simulink model "cranePoleMDL"  (R2014a)
settings: Solver=ode45  StartTime=0.0  StopTime=10.0  RelTol=1e-3
values from neighbouring files (symbols this model uses):
  F = A1-K1*C    [cartPole.m]    (also in chenEx3p3p3.m = A1-k1*C)
  g = 9.8    [cartPole.m]
  K = K1 + F*H    [cartPole.m]
  l = 0.3    [cartPole.m]
  M = .5    (= 0.5)    [cartPole.m]
  m = .2    (= 0.2)    [cartPole.m]
  theta_0 = pi    (= 3.14159265359)    [cartPole.m]
  theta_d_0 = 0.0    (= 0)    [cartPole.m]
  x1_0 = -1    [chenEx3p3p3.m]
  x3_0 = 1    [chenEx3p3p3.m]
  x_0 = 0    [cartPole.m]
  x_d_0 = 0    [cartPole.m]
undefined symbols (not defined in the file or in its folder): Klqr
settings Model: Creator=sqn4594  LastModifiedBy=sqn4594

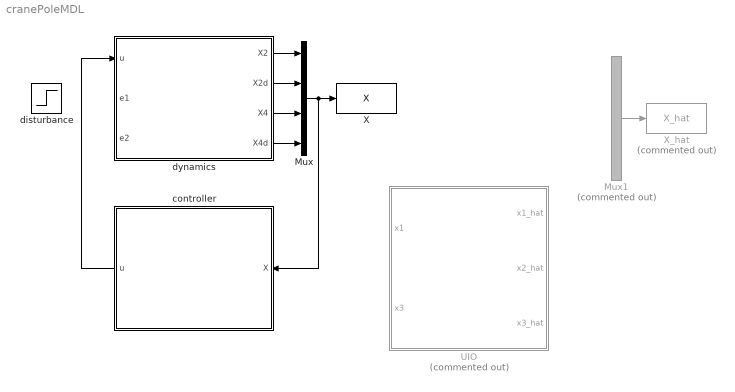
== system cranePoleMDL ==
  Mux : Mux
  Mux1 : Mux  Commented=on  Inputs=3
  UIO : Subsystem  Commented=on
  X : ToWorkspace  VariableName=X  SampleTime=-1
  X_hat : ToWorkspace  Commented=on  VariableName=X_hat  SampleTime=-1
  controller : Subsystem
  disturbance : Step  After=1e-3  SampleTime=0
  dynamics : Subsystem
  wires:
  Mux/1 -> controller/1(X), X/1
  Mux1/1 -> X_hat/1
  dynamics/2(X2d) -> Mux/2
  dynamics/4(X4d) -> Mux/4
  dynamics/1("X2 ") -> Mux/1
  dynamics/3("X4 ") -> Mux/3
  controller/1(u) -> dynamics/1(u)

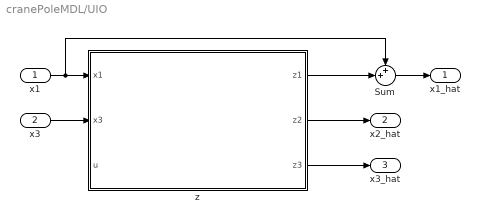
== system cranePoleMDL/UIO ==
  x1 : Inport
  x3 : Inport  Port=2
  Sum : Sum  Inputs=++|
  z : Subsystem
  x1_hat : Outport
  x2_hat : Outport  Port=2
  x3_hat : Outport  Port=3
  wires:
  x1/1 -> Sum/1, z/1(x1)
  x3/1 -> z/2(x3)
  z/1(z1) -> Sum/2
  Sum/1 -> x1_hat/1
  z/2(z2) -> x2_hat/1
  z/3(z3) -> x3_hat/1

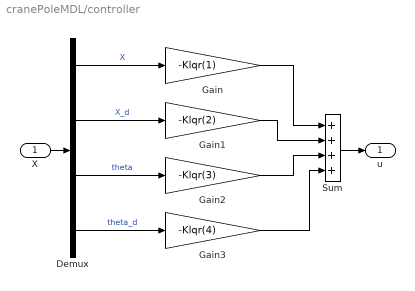
== system cranePoleMDL/controller ==
  X : Inport
  Demux : Demux
  Gain : Gain  Gain=-Klqr(1)
  Gain1 : Gain  Gain=-Klqr(2)
  Gain2 : Gain  Gain=-Klqr(3)
  Gain3 : Gain  Gain=-Klqr(4)
  Sum : Sum  Inputs=++++
  u : Outport
  wires:
  X/1 -> Demux/1
  Demux/1 -> Gain/1  "X"
  Demux/2 -> Gain1/1  "X_d"
  Demux/3 -> Gain2/1  "theta"
  Demux/4 -> Gain3/1  "theta_d"
  Sum/1 -> u/1
  Gain/1 -> Sum/1
  Gain1/1 -> Sum/2
  Gain2/1 -> Sum/3
  Gain3/1 -> Sum/4

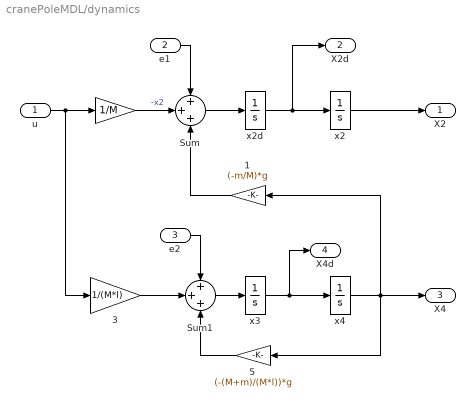
== system cranePoleMDL/dynamics ==
  u : Inport
  e1 : Inport  Port=2
  e2 : Inport  Port=3
  "  " : Gain  Gain=1/M
  "  1" : Gain  Gain=(-m/M)*g
  "  3" : Gain  Gain=1/(M*l)
  "  5" : Gain  Gain=(-(M+m)/(M*l))*g
  Sum : Sum  Inputs=+++
  Sum1 : Sum  Inputs=+++
  x2 : Integrator  InitialCondition=x_0
  x2d : Integrator  InitialCondition=x_d_0
  x3 : Integrator  InitialCondition=theta_d_0
  x4 : Integrator  InitialCondition=theta_0
  "X2 " : Outport
  X2d : Outport  Port=2
  "X4 " : Outport  Port=3
  X4d : Outport  Port=4
  wires:
  u/1 -> "  3"/1, "  "/1
  e1/1 -> Sum/1
  Sum/1 -> x2d/1
  x2d/1 -> X2d/1, x2/1
  Sum1/1 -> x3/1
  "  3"/1 -> Sum1/2
  x2/1 -> "X2 "/1
  x4/1 -> "  1"/1, "  5"/1, "X4 "/1
  x3/1 -> X4d/1, x4/1
  "  "/1 -> Sum/2  "-x2"
  e2/1 -> Sum1/1
  "  5"/1 -> Sum1/3
  "  1"/1 -> Sum/3

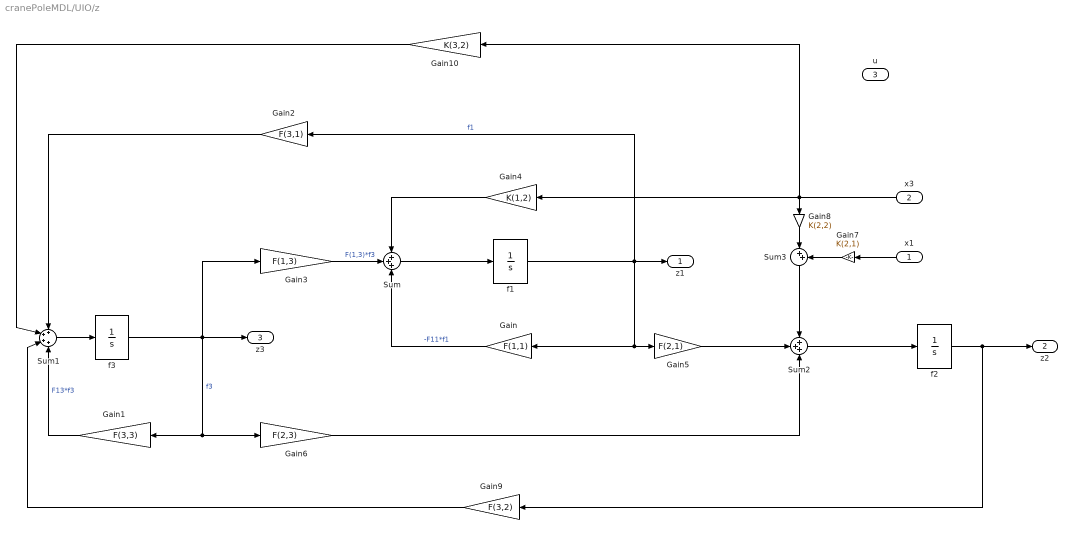
== system cranePoleMDL/UIO/z ==
  x1 : Inport
  x3 : Inport  Port=2
  u : Inport  Port=3
  Gain : Gain  Gain=F(1,1)
  Gain1 : Gain  Gain=F(3,3)
  Gain10 : Gain  Gain=K(3,2)
  Gain2 : Gain  Gain=F(3,1)
  Gain3 : Gain  Gain=F(1,3)
  Gain4 : Gain  Gain=K(1,2)
  Gain5 : Gain  Gain=F(2,1)
  Gain6 : Gain  Gain=F(2,3)
  Gain7 : Gain  Gain=K(2,1)
  Gain8 : Gain  Gain=K(2,2)
  Gain9 : Gain  Gain=F(3,2)
  Sum : Sum  Inputs=+++
  Sum1 : Sum  Inputs=++++
  Sum2 : Sum  Inputs=+++
  Sum3 : Sum  Inputs=|++
  f1 : Integrator  InitialCondition=x1_0
  f2 : Integrator  InitialCondition=x1_0
  f3 : Integrator  InitialCondition=x3_0
  z1 : Outport
  z2 : Outport  Port=2
  z3 : Outport  Port=3
  wires:
  Sum2/1 -> f2/1
  Sum3/1 -> Sum2/1
  f2/1 -> z2/1, Gain9/1
  x3/1 -> Gain10/1, Gain8/1, Gain4/1
  Gain10/1 -> Sum1/2
  Gain9/1 -> Sum1/3
  Gain2/1 -> Sum1/1
  Gain/1 -> Sum/3  "-F11*f1"
  Gain6/1 -> Sum2/3
  Gain5/1 -> Sum2/2
  Gain4/1 -> Sum/1
  Gain7/1 -> Sum3/2
  x1/1 -> Gain7/1
  Gain3/1 -> Sum/2  "F(1,3)*f3"
  Gain8/1 -> Sum3/1
  Sum/1 -> f1/1
  f1/1 -> z1/1, Gain5/1, Gain/1, Gain2/1  "f1"
  Gain1/1 -> Sum1/4  "F13*f3"
  Sum1/1 -> f3/1
  f3/1 -> z3/1, Gain3/1, Gain1/1, Gain6/1  "f3"
